simulink model "eVTOL_PX4_2023b"  (R2024b)
settings: Solver=ode4  StartTime=0  StopTime=inf  FixedStep=0.01  RelTol=1e-3
values from neighbouring files (symbols this model uses):
  aDl =     [initdata.mat]
  aDr =     [initdata.mat]
  aDyn =     [initdata.mat]
  Airport = init_airport('PHNL')    [initdata_HIL_eVTOL.m]
  aLat =     [initdata.mat]
  aLon =     [initdata.mat]
  D = Prop.D    [EOM_dt_MC.m]    (also in EOM_get_alf_dt_de_prop_evtol.m = CD * QS)
  dt0 = X(2)    [EOM_get_alf_dt_de_prop_evtol.m]    (also in initdata.mat = 0.258252593971; initdata_HIL_eVTOL.m = EOM_dt_MC)
  EAS0 = TAS0 / EAS2TAS    [initdata_HIL_eVTOL.m]
  FCS = init_FCS    [initdata_HIL_eVTOL.m]
  General = init_layoutdata    [EOM_dt_MC.m]    (also in build_optimized_CA.m; initdata.mat = ; initdata_HIL_eVTOL.m)
  h0 = Con(1)    [EOM_get_alf_dt_de_prop_evtol.m]    (also in initdata.mat = 450; initdata_HIL_eVTOL.m = 50)
  mass = Con(3)    [EOM_get_alf_dt_de_prop_evtol.m]    (also in initdata.mat = 2255.54; initdata_HIL_eVTOL.m = 7)
  Motor = init_motor_evtol    [EOM_dt_MC.m]    (also in initdata.mat = []; initdata_HIL_eVTOL.m)
  Prop = init_propeller_evtol_new    [EOM_dt_MC.m]    (also in initdata_HIL_eVTOL.m)
  R2D = 180/pi    (= 57.2957795131)    [EOM_get_alf_dt_de_prop_evtol.m]    (also in init_FCS.m; init_aerodata_evtol.m; init_airport.m; initdata.mat)
  SAMPLE_TIME = 0.01    [initdata_HIL_eVTOL.m]
  theta0 = -0.0510981441662    [initdata.mat]
undefined symbols (not defined in the file or in its folder): A1, aDa, aDe, aero, asbhl20env, B1, C1, de0, Earth, Environment, INIT_Data, InitData, Kd, Kp, magnitude, Newton, pProp, Raphson, Tc, WGS84
libraries: simulink_extras x63, vrlib x48, sharedtransform x28, simulink x22, slpidlib x20, sharedutil x20, matrix_library x18, aerolibwindfilters x12, aerolibobsolete x8, aerolibasang x8, aerolibatmos2 x6, aerolibfltsims x6
(part 7 of 17)

== system eVTOL_PX4_2023b/Subsystem2/Environment/Wind Models ==
  Xe_x : Inport
  Ve : Inport  Port=2
  Altitude : Inport  Port=3
  DCM : Inport  Port=4
  Constant1 : Constant  Value=[0,0,0]
  Constant2 : Constant  Value=[0,0,0]
  Dot Product1 : DotProduct  OutDataTypeStr=Inherit: Inherit via internal rule
  Dot Product2 : DotProduct  OutDataTypeStr=Inherit: Inherit via internal rule
  Dryden Wind Turbulence Model (Continuous (+q -r)) : Subsystem  AncestorBlock=|  mask(Wind Turbulence Model){units=Metric (MKS), spec=MIL-F-8785C, model=Continuous Dryden (+q -r), W20=8, Wdeg=0, TurbProb=10^-4, L_high=533.4, Wingspan=7, ts=0.01, Seed=[23341 23342 23343 23344], T_on=on}
      | CustomLib_2019b/Dryden Wind Turbulence Model 
      | (Continuous (+q -r))
      mask prompts: units "aeroblks:aeroblkwind:blockWindTurbulenceModelParamUnits"; spec "aeroblks:aeroblkwind:blockWindTurbulenceModelParamSpecification"; model "aeroblks:aeroblkwind:blockWindTurbulenceModelParamModeltype"; W20 "Wind speed at 6 m defines the low-altitude intensity (m/s):"; Wdeg "Wind direction at 6 m (degrees clockwise from north):"; TurbProb "aeroblks:aeroblkwind:blockWindTurbulenceModelParamProbabilityofexceedanceofhighaltitudeintensity"; L_high "Scale length at medium/high altitudes (m):"; Wingspan "Wingspan (m):"; ts "Band limited noise sample time (sec):"; Seed "aeroblks:aeroblkwind:blockWindTurbulenceModelParamNoiseseedsugvgwgpg"; T_on "aeroblks:aeroblkwind:blockWindTurbulenceModelParamTurbulenceon"
      mask help: aeroblks:aeroblkwind:blockWindTurbulenceModelDesc
      mask init: same as eVTOL_PX4_2023b/Subsystem1/Environment/Wind Models/Dryden Wind Turbulence Model (Continuous (+q -r))
      settings: LibrarySourceBlock=|
      | CustomLib_2019b/Dryden Wind Turbulence Model
      | (Continuous (+q -r))
      mask Help: eval('asbhelp(''Dryden Wind Turbulence Model (Continuous)'')');
      mask TypeOptions units: aeroblks:aeroblkwind:blockWindTurbulenceModelParamComboMetricMKS | aeroblks:aeroblkwind:blockWindTurbulenceModelParamComboEnglishVelocityinfts | aeroblks:aeroblkwind:blockWindTurbulenceModelParamComboEnglishVelocityinkts
      mask TypeOptions spec: aeroblks:aeroblkwind:blockWindTurbulenceModelParamComboMILF8785C | aeroblks:aeroblkwind:blockWindTurbulenceModelParamComboMILHDBK1797 | aeroblks:aeroblkwind:blockWindTurbulenceModelParamComboMILHDBK1797B
      mask TypeOptions model: aeroblks:aeroblkwind:blockWindTurbulenceModelParamComboContinuousVonKarmanqr1 | aeroblks:aeroblkwind:blockWindTurbulenceModelParamComboContinuousVonKarmanqr2 | aeroblks:aeroblkwind:blockWindTurbulenceModelParamComboContinuousVonKarmanqr3 | aeroblks:aeroblkwind:blockWindTurbulenceModelParamComboContinuousDrydenqr1 | aeroblks:aeroblkwind:blockWindTurbulenceModelParamComboContinuousDrydenqr2 | aeroblks:aeroblkwind:blockWindTurbulenceModelParamComboContinuousDrydenqr3 | aeroblks:aeroblkwind:blockWindTurbulenceModelParamComboDiscreteDrydenqr1 | aeroblks:aeroblkwind:blockWindTurbulenceModelParamComboDiscreteDrydenqr2 | aeroblks:aeroblkwind:blockWindTurbulenceModelParamComboDiscreteDrydenqr3
      mask Callback model: aeroicon('aeroblkwindturb2');
      mask TypeOptions TurbProb: aeroblks:aeroblkwind:blockWindTurbulenceModelParamCombo2x101 | aeroblks:aeroblkwind:blockWindTurbulenceModelParamCombo101 | aeroblks:aeroblkwind:blockWindTurbulenceModelParamCombo102Light | aeroblks:aeroblkwind:blockWindTurbulenceModelParamCombo103Moderate | aeroblks:aeroblkwind:blockWindTurbulenceModelParamCombo104 | aeroblks:aeroblkwind:blockWindTurbulenceModelParamCombo105Severe | aeroblks:aeroblkwind:blockWindTurbulenceModelParamCombo106
      mask DialogControl units Prompt: Units:
      mask DialogControl spec Prompt: Specification:
      mask DialogControl model Prompt: Model type:
      mask DialogControl TurbProb Prompt: Probability of exceedance of high-altitude intensity:
      mask DialogControl Seed Prompt: Noise seeds [ug vg wg pg]:
      mask DialogControl T_on Prompt: Turbulence on
      mask Display:
      | port_label(ports(1).type,ports(1).port,ports(1).txt,'texmode','on');
      | port_label(ports(2).type,ports(2).port,ports(2).txt,'texmode','on');
      | port_label(ports(3).type,ports(3).port,ports(3).txt,'texmode','on');
      | port_label(ports(4).type,ports(4).port,ports(4).txt,'texmode','on');
      | port_label(ports(5).type,ports(5).port,ports(5).txt,'texmode','on');
  Gain4 : Gain  Gain=[1,1,1]
  Manual Switch1 : ManualSwitch  CurrentSetting=0
  Manual Switch2 : ManualSwitch  CurrentSetting=0
  Sqrt : Sqrt
  vt1 : Math  Operator=sqrt  SignedPower=on
  wind scp2 : Scope
  wind_mag scp : Scope
  windangular scp : Scope
  windspeed scp : Scope
  ug,vg,wg1 : Outport  VectorParamsAs1DForOutWhenUnconnected=off
  pg,qg,rg1 : Outport  Port=2  VectorParamsAs1DForOutWhenUnconnected=off
  wires:
  Manual Switch2/1 -> ug,vg,wg1/1  "WindVelocity"
  Dryden Wind Turbulence Model (Continuous (+q -r))/1(ug,vg,wg) -> Gain4/1, windspeed scp/1, Dot Product2/2, Dot Product2/1  "Vw"
  Dryden Wind Turbulence Model (Continuous (+q -r))/2(pg,qg,rg) -> Manual Switch1/1, windangular scp/1  "WindAngularRates"
  Constant1/1 -> Manual Switch1/2
  Altitude/1 -> [Altitude]
  vt1/1 -> [Airspeed]  "Airspeed"
  Constant2/1 -> Manual Switch2/2
  [Airspeed] -> Dryden Wind Turbulence Model (Continuous (+q -r))/2(Airspeed)  "Airspeed"
  DCM/1 -> [DCM]
  Ve/1 -> Dot Product1/2, Dot Product1/1
  Manual Switch1/1 -> pg,qg,rg1/1  "WindAngularRates"
  Gain4/1 -> Manual Switch2/1  "WindVelocity"
  [Altitude] -> Dryden Wind Turbulence Model (Continuous (+q -r))/1(Altitude)
  Dot Product2/1 -> Sqrt/1
  [DCM] -> Dryden Wind Turbulence Model (Continuous (+q -r))/3(DCM)
  Dot Product1/1 -> vt1/1
  Sqrt/1 -> wind_mag scp/1  "wind_mag"
  Xe_x/1 -> [x]
  [x] -> wind scp2/1

== system eVTOL_PX4_2023b/Subsystem2/airframe/Flight Conditions ==
  EnvmData : Inport
  PlantData : Inport  Port=2
  Bus Selector1 : BusSelector  OutputSignals=WindVelocity,a,AirDensity,WindAngularRates,Po,To,g
  Bus Selector2 : BusSelector  OutputSignals=Xe,Ve,Vb,pqr,DCM_be
  Constant1 : Constant  Value=Airport.Elevation_m
  Constant2 : Constant  Value=1.225
  Demux : Demux  Outputs=2
  Derivative : Derivative  CoefficientInTFapproximation=100
  Divide : Product  Inputs=*/
  Divide1 : Product  Inputs=**
  Dynamic Pressure : aerolibasang/Dynamic Pressure
  Flat Earth to LLA1 : aerolibtransform2/Flat Earth to LLA  units=Metric (MKS)  ptype=Earth (WGS84)  F=1/298.257223563  R=6378137  refPosPort=off  LL0=InitData.LLA(1:2)*R2D  psi=0
  "Incidence, Sideslip, & Airspeed" : Subsystem  AncestorBlock=aerolibasang/Incidence, Sideslip, & Airspeed  mask(Incidence,Sideslip,&Airspeed){}
      mask help: Calculate the angles between the body and the velocity vector (incidence and sideslip), and the velocity magnitude from the components in body axes (Vb).
      settings: LibrarySourceBlock=|
      | aerolibasang/Incidence, Sideslip,
      | & Airspeed
      mask Help: web(asbhelp('incidence'));
      mask Display:
      | port_label('input',1,'V_b','texmode','on');
      | port_label('output',1,'\alpha','texmode','on');
      | port_label('output',2,'\beta','texmode','on');
      | port_label('output',3,'V','texmode','on');
  Mach Number : aerolibasang/Mach Number
  Product : Product  Multiplication=Matrix(*)
  Product1 : Product  Multiplication=Matrix(*)
  Sqrt : Sqrt
  Subsystem : Subsystem
  Sum1 : Sum  Inputs=+-|  InputSameDT=on  SaturateOnIntegerOverflow=on  OutDataTypeStr=Inherit: Same as first input
  Sum2 : Sum  Inputs=|+-  InputSameDT=on  SaturateOnIntegerOverflow=on  OutDataTypeStr=Inherit: Same as first input
  Terminator : Terminator
  Vw_b : Scope
  Vw_e : Scope
  lat_deg : Outport  VectorParamsAs1DForOutWhenUnconnected=off
  lon_deg : Outport  Port=2  VectorParamsAs1DForOutWhenUnconnected=off
  amsl : Outport  Port=3  VectorParamsAs1DForOutWhenUnconnected=off
  Alpha : Outport  Port=4  VectorParamsAs1DForOutWhenUnconnected=off
  AlphaDot : Outport  Port=5  VectorParamsAs1DForOutWhenUnconnected=off
  Beta : Outport  Port=6  VectorParamsAs1DForOutWhenUnconnected=off
  V : Outport  Port=7  VectorParamsAs1DForOutWhenUnconnected=off
  EAS : Outport  Port=8  VectorParamsAs1DForOutWhenUnconnected=off
  pqrWind : Outport  Port=9  VectorParamsAs1DForOutWhenUnconnected=off
  Mach : Outport  Port=10  VectorParamsAs1DForOutWhenUnconnected=off
  Qbar : Outport  Port=11  InitialOutput=0  VectorParamsAs1DForOutWhenUnconnected=off
  gamma : Outport  Port=12  InitialOutput=0  VectorParamsAs1DForOutWhenUnconnected=off
  chi : Outport  Port=13  InitialOutput=0  VectorParamsAs1DForOutWhenUnconnected=off
  Po : Outport  Port=14  VectorParamsAs1DForOutWhenUnconnected=off
  To : Outport  Port=15  VectorParamsAs1DForOutWhenUnconnected=off
  g : Outport  Port=16  VectorParamsAs1DForOutWhenUnconnected=off
  wires:
  Derivative/1 -> AlphaDot/1
  Bus Selector1/4 -> Product1/2  "<WindAngularRates>"
  Subsystem/1(gamma) -> gamma/1
  PlantData/1 -> Bus Selector2/1
  Sum2/1 -> "Incidence, Sideslip, & Airspeed"/1(Vb), Mach Number/1, Dynamic Pressure/1  "VA(b)"
  Subsystem/2(chi) -> chi/1
  Bus Selector2/3 -> Sum2/1  "<Vb>"
  Subsystem/3(V) -> Terminator/1
  Product1/1 -> Sum1/2
  Bus Selector1/5 -> Po/1  "<Po>"
  Mach Number/1 -> Mach/1  "Mach"
  "Incidence, Sideslip, & Airspeed"/1(Alpha) -> Derivative/1, Alpha/1  "Alpha"
  Product/1 -> Vw_b/1, Sum2/2
  Bus Selector2/2 -> Subsystem/1(<Ve>)  "<Ve>"
  "Incidence, Sideslip, & Airspeed"/2(Beta) -> Beta/1  "Beta"
  Dynamic Pressure/1 -> Qbar/1  "qbar"
  Bus Selector1/2 -> Mach Number/2  "<a>"
  Bus Selector2/5 -> Product/1, Product1/1  "<DCM_be>"
  Bus Selector2/4 -> Sum1/1  "<pqr>"
  Sum1/1 -> pqrWind/1
  EnvmData/1 -> Bus Selector1/1
  Bus Selector1/3 -> Divide/1, Dynamic Pressure/2  "<AirDensity>"
  Bus Selector1/1 -> Product/2, Vw_e/1  "<WindVelocity>"
  Bus Selector1/7 -> g/1  "<g>"
  Bus Selector1/6 -> To/1  "<To>"
  Demux/1 -> lat_deg/1  "lat_deg"
  Demux/2 -> lon_deg/1  "lon_deg"
  Flat Earth to LLA1/2 -> amsl/1  "amsl"
  Flat Earth to LLA1/1 -> Demux/1
  Constant1/1 -> Flat Earth to LLA1/2
  Bus Selector2/1 -> Flat Earth to LLA1/1  "<Xe>"
  Constant2/1 -> Divide/2
  Divide1/1 -> EAS/1
  Divide/1 -> Sqrt/1
  "Incidence, Sideslip, & Airspeed"/3(V) -> Divide1/1, V/1  "V"
  Sqrt/1 -> Divide1/2

== system eVTOL_PX4_2023b/Subsystem2/airframe/force moment ==
  note: force and moment in body fixed axis coordination
  PlantData : Inport
  Act_surface : Inport  Port=2
  prop : Inport  Port=3
  EnvmData : Inport  Port=4
  Add : Sum  Inputs=++++
  Add1 : Sum  Inputs=++++
  Disturbance : Constant  Value=[0,10,0]
  Disturbance1 : Constant  Value=[0,0,0]
  F_Gear_in_b scp : Scope  Commented=on
  Gear&FM in body axis : Subsystem  Commented=on
  M_Gear scp : Scope  Commented=on
  Manual Switch : ManualSwitch  CurrentSetting=0
  Motor moment scp : Scope
  Scope{,1..4,6} (6 alike) : Scope
  Thrust&M in body axis : Subsystem
  aero F&M in body axis : Subsystem
  gravity in body axis : Subsystem
  Fb (X Y Z) : Outport  VectorParamsAs1DForOutWhenUnconnected=off
  M (L M N) : Outport  Port=2  VectorParamsAs1DForOutWhenUnconnected=off
  wires:
  Thrust&M in body axis/1(f_T) -> Add/1, Scope4/1
  gravity in body axis/1(Fb) -> Add/3, Scope3/1
  Thrust&M in body axis/2(m_T) -> Add1/1, Motor moment scp/1
  aero F&M in body axis/2(M (L M N)) -> Scope6/1, Add1/2
  Add1/1 -> Scope1/1, M (L M N)/1
  Add/1 -> Scope/1, Fb (X Y Z)/1
  PlantData/1 -> aero F&M in body axis/1(PlantData), Gear&FM in body axis/1(PlantData), gravity in body axis/1(PlantData)
  Act_surface/1 -> aero F&M in body axis/2(Act_surface)
  EnvmData/1 -> gravity in body axis/2(EnvmData)
  Gear&FM in body axis/1(F_Gear) -> Add/4, F_Gear_in_b scp/1
  Gear&FM in body axis/2(M_Gear) -> Add1/3, M_Gear scp/1
  aero F&M in body axis/1(Fb (X Y Z)) -> Add/2, Scope2/1
  Disturbance/1 -> Manual Switch/1
  Manual Switch/1 -> Add1/4
  Disturbance1/1 -> Manual Switch/2
  prop/1 -> Thrust&M in body axis/1(prop)

== system eVTOL_PX4_2023b/UAV/Environment/Terrain ==
  Xe : Inport
  Terminator : Terminator
  hground_value : Constant  OutDataTypeStr=single
  hground : Outport  VectorParamsAs1DForOutWhenUnconnected=off
  wires:
  Xe/1 -> Terminator/1
  hground_value/1 -> hground/1  "hground"

== system eVTOL_PX4_2023b/UAV/Environment/Wind Models ==
  WindSpeed : Inport
  Ve : Inport  Port=2
  Altitude : Inport  Port=3
  DCM : Inport  Port=4
  Constant : Constant  Value=0
  Discrete Wind Gust Model1 : aerolibwind2/Discrete Wind Gust Model  units=Metric (MKS)  Gx=on  Gy=off  Gz=off  t_0=20  d_m=[10 10 6]*4  v_m=-[3.5 3.5 2.0]*1
  Discrete Wind Gust Model2 : aerolibwind2/Discrete Wind Gust Model  units=Metric (MKS)  Gx=on  Gy=off  Gz=off  t_0=28  d_m=[10 10 6]*4  v_m=[3.5 3.5 2.0]*1
  Dot Product : DotProduct  OutDataTypeStr=Inherit: Inherit via internal rule
  Gain : Gain
  Manual Switch : ManualSwitch
  Mux : Mux  Inputs=3
  Pulse Generator : DiscretePulseGenerator  PulseType=Time based  Amplitude=5  Period=1000  PulseWidth=99  PhaseDelay=1
  Sine Wave : Sin  Amplitude=0.2  SampleTime=0
  Sum : Sum  Inputs=+++++  InputSameDT=on  SaturateOnIntegerOverflow=on  OutDataTypeStr=Inherit: Same as first input
  Sum1 : Sum  Inputs=|++
  To Workspace8 : ToWorkspace  VariableName=VWindscp  SampleTime=-1
  Transform from Inertial to Body axes : Product  Inputs=**  Multiplication=Matrix(*)  InputSameDT=on  SaturateOnIntegerOverflow=on  OutDataTypeStr=Inherit: Same as first input
  constance wind : Constant  Value=[0, 2, 1]
  constance wind1 : Constant  Value=[0, 0, 0]
  constance wind2 : Constant  Value=[0, -2, 0]
  vt : Math  Operator=sqrt  SignedPower=on
  wind scp : Scope
  ug,vg,wg : Outport  VectorParamsAs1DForOutWhenUnconnected=off
  pg,qg,rg : Outport  Port=2  VectorParamsAs1DForOutWhenUnconnected=off
  wires:
  Ve/1 -> Dot Product/2, Dot Product/1
  Dot Product/1 -> vt/1
  vt/1 -> [Airspeed]  "Airspeed"
  Altitude/1 -> [Altitude]
  DCM/1 -> [DCM]
  Sum/1 -> To Workspace8/1, wind scp/1, ug,vg,wg/1  "WindVelocity"
  ? -> Sum/3
  [Airspeed] -> Discrete Wind Gust Model2/1, Discrete Wind Gust Model1/1  "Airspeed"
  constance wind1/1 -> pg,qg,rg/1  "WindAngularRates"
  [Altitude] -> ?
  [DCM] -> ?
  [Altitude] -> ?
  constance wind/1 -> ?
  [DCM] -> Transform from Inertial to Body axes/1
  Transform from Inertial to Body axes/1 -> Sum/1
  Constant/1 -> ?
  Mux/1 -> Manual Switch/2
  Manual Switch/1 -> Transform from Inertial to Body axes/2
  Sine Wave/1 -> Mux/3, Mux/2, Mux/1
  constance wind2/1 -> ?
  Discrete Wind Gust Model2/1 -> Sum1/2
  Sum1/1 -> Gain/1
  Discrete Wind Gust Model1/1 -> Sum1/1
  Gain/1 -> ?
  WindSpeed/1 -> Manual Switch/1

== system eVTOL_PX4_2023b/UAV/airframe/Flight Conditions ==
  EnvmData : Inport
  PlantData : Inport  Port=2
  Bus Selector1 : BusSelector  OutputSignals=WindVelocity,a,AirDensity,WindAngularRates,Po,To,g
  Bus Selector2 : BusSelector  OutputSignals=Xe,Ve,Vb,pqr
  Constant : Constant  Value=0
  Constant1 : Constant  Value=1.225
  Demux : Demux  Outputs=2
  Divide : Product  Inputs=*/
  Divide1 : Product  Inputs=**
  Dynamic Pressure : aerolibasang/Dynamic Pressure
  Flat Earth to LLA : aerolibtransform2/Flat Earth to LLA  units=Metric (MKS)  ptype=Earth (WGS84)  F=1/298.257223563  R=6378137  refPosPort=off  LL0=[INIT_Data.lat_deg, INIT_Data.lon_deg]  psi=0
  "Incidence, Sideslip, & Airspeed" : Subsystem  AncestorBlock=aerolibasang/Incidence, Sideslip, & Airspeed  mask(Incidence,Sideslip,&Airspeed){}
      mask help: Calculate the angles between the body and the velocity vector (incidence and sideslip), and the velocity magnitude from the components in body axes (Vb).
      mask Help: web(asbhelp('incidence'));
      mask Display:
      | port_label('input',1,'V_b','texmode','on');
      | port_label('output',1,'\alpha','texmode','on');
      | port_label('output',2,'\beta','texmode','on');
      | port_label('output',3,'V','texmode','on');
  Mach Number : aerolibasang/Mach Number
  Selector : Selector  InputPortWidth=3  IndexOptions=Index vector (dialog)  Indices=2  OutputSizes=1
  Sqrt : Sqrt
  Subsystem : Subsystem
  Sum1 : Sum  Inputs=++|  InputSameDT=on  SaturateOnIntegerOverflow=on  OutDataTypeStr=Inherit: Same as first input
  Sum2 : Sum  Inputs=|+-  InputSameDT=on  SaturateOnIntegerOverflow=on  OutDataTypeStr=Inherit: Same as first input
  Terminator : Terminator
  lat_deg : Outport  VectorParamsAs1DForOutWhenUnconnected=off
  lon_deg : Outport  Port=2  VectorParamsAs1DForOutWhenUnconnected=off
  amsl : Outport  Port=3  VectorParamsAs1DForOutWhenUnconnected=off
  Alpha : Outport  Port=4  VectorParamsAs1DForOutWhenUnconnected=off
  AlphaDot : Outport  Port=5  VectorParamsAs1DForOutWhenUnconnected=off
  Beta : Outport  Port=6  VectorParamsAs1DForOutWhenUnconnected=off
  V : Outport  Port=7  VectorParamsAs1DForOutWhenUnconnected=off
  EAS : Outport  Port=8  VectorParamsAs1DForOutWhenUnconnected=off
  pqrWind : Outport  Port=9  VectorParamsAs1DForOutWhenUnconnected=off
  Mach : Outport  Port=10  VectorParamsAs1DForOutWhenUnconnected=off
  Qbar : Outport  Port=11  InitialOutput=0  VectorParamsAs1DForOutWhenUnconnected=off
  gamma : Outport  Port=12  InitialOutput=0  VectorParamsAs1DForOutWhenUnconnected=off
  chi : Outport  Port=13  InitialOutput=0  VectorParamsAs1DForOutWhenUnconnected=off
  Po : Outport  Port=14  VectorParamsAs1DForOutWhenUnconnected=off
  To : Outport  Port=15  VectorParamsAs1DForOutWhenUnconnected=off
  g : Outport  Port=16  VectorParamsAs1DForOutWhenUnconnected=off
  wires:
  "Incidence, Sideslip, & Airspeed"/2(Beta) -> Beta/1  "Beta"
  "Incidence, Sideslip, & Airspeed"/3(V) -> Divide1/1, V/1  "V"
  Mach Number/1 -> Mach/1  "Mach"
  Dynamic Pressure/1 -> Qbar/1  "qbar"
  PlantData/1 -> Bus Selector2/1
  EnvmData/1 -> Bus Selector1/1
  Sum2/1 -> "Incidence, Sideslip, & Airspeed"/1(Vb), Mach Number/1, Dynamic Pressure/1  "VA(b)"
  Bus Selector2/3 -> Sum2/1  "<Vb>"
  Bus Selector1/1 -> Sum2/2  "<WindVelocity>"
  Bus Selector1/2 -> Mach Number/2  "<a>"
  Bus Selector1/3 -> [rho]  "<AirDensity>"
  Bus Selector1/4 -> Sum1/2  "<WindAngularRates>"
  Bus Selector2/4 -> [pqr]  "<pqr>"
  Sum1/1 -> pqrWind/1
  "Incidence, Sideslip, & Airspeed"/1(Alpha) -> Alpha/1  "Alpha"
  Selector/1 -> AlphaDot/1
  Bus Selector2/2 -> Subsystem/1(Xe)  "<Ve>"
  Subsystem/1(chi) -> chi/1
  Subsystem/2(gamma) -> gamma/1
  Subsystem/3(R) -> Terminator/1
  Bus Selector1/6 -> To/1  "<To>"
  Bus Selector1/5 -> Po/1  "<Po>"
  Bus Selector1/7 -> g/1  "<g>"
  Flat Earth to LLA/2 -> amsl/1  "amsl"
  Demux/1 -> lat_deg/1  "lat_deg"
  Demux/2 -> lon_deg/1  "lon_deg"
  Constant/1 -> Flat Earth to LLA/2
  Flat Earth to LLA/1 -> Demux/1
  Bus Selector2/1 -> Flat Earth to LLA/1  "<Xe>"
  [pqr] -> Sum1/1
  [pqr] -> Selector/1
  [rho] -> Dynamic Pressure/2
  [rho] -> Divide/1
  Constant1/1 -> Divide/2
  Divide/1 -> Sqrt/1
  Sqrt/1 -> Divide1/2
  Divide1/1 -> EAS/1

== system eVTOL_PX4_2023b/UAV/airframe/force moment ==
  note: force and moment in body fixed axis coordination
  PlantData : Inport
  ActData : Inport  Port=2
  EngineData_lo : Inport  Port=3
  EnvmData : Inport  Port=4
  Add : Sum  Inputs=++++
  Add1 : Sum  Inputs=++++
  Disturbance : Constant  Value=[0,10,0]
  Disturbance1 : Constant  Value=[0,0,0]
  F_Gear_in_b scp : Scope
  Gear&FM in body axis : Subsystem  Commented=on
  Gear&FM in body axis1 : Subsystem
  M_Gear scp : Scope
  Manual Switch : ManualSwitch  CurrentSetting=0
  Motor moment scp : Scope
  Scope{,1..4,6} (6 alike) : Scope
  Thrust in body axis1 : Subsystem
  aero F&M in body axis : Subsystem
  gravity in body axis : Subsystem
  Fb (X Y Z) : Outport  VectorParamsAs1DForOutWhenUnconnected=off
  M (L M N) : Outport  Port=2  VectorParamsAs1DForOutWhenUnconnected=off
  wires:
  Thrust in body axis1/1(f_T) -> Add/1, Scope4/1
  gravity in body axis/1(Fb) -> Add/3, Scope3/1
  Thrust in body axis1/2(m_T) -> Add1/1, Motor moment scp/1
  aero F&M in body axis/2(M (L M N)) -> Add1/2, Scope6/1
  Add1/1 -> M (L M N)/1, Scope1/1
  Add/1 -> Fb (X Y Z)/1, Scope/1
  PlantData/1 -> aero F&M in body axis/1(PlantData), Gear&FM in body axis1/1(PlantData), gravity in body axis/1(PlantData)
  ActData/1 -> aero F&M in body axis/2(ActData)
  EngineData_lo/1 -> Thrust in body axis1/1(EngineData)
  EnvmData/1 -> gravity in body axis/2(EnvmData)
  Gear&FM in body axis1/1(F_Gear) -> Add/4, F_Gear_in_b scp/1
  Gear&FM in body axis1/2(M_Gear) -> Add1/3, M_Gear scp/1
  aero F&M in body axis/1(Fb (X Y Z)) -> Add/2, Scope2/1
  Disturbance/1 -> Manual Switch/1
  Manual Switch/1 -> Add1/4
  Disturbance1/1 -> Manual Switch/2

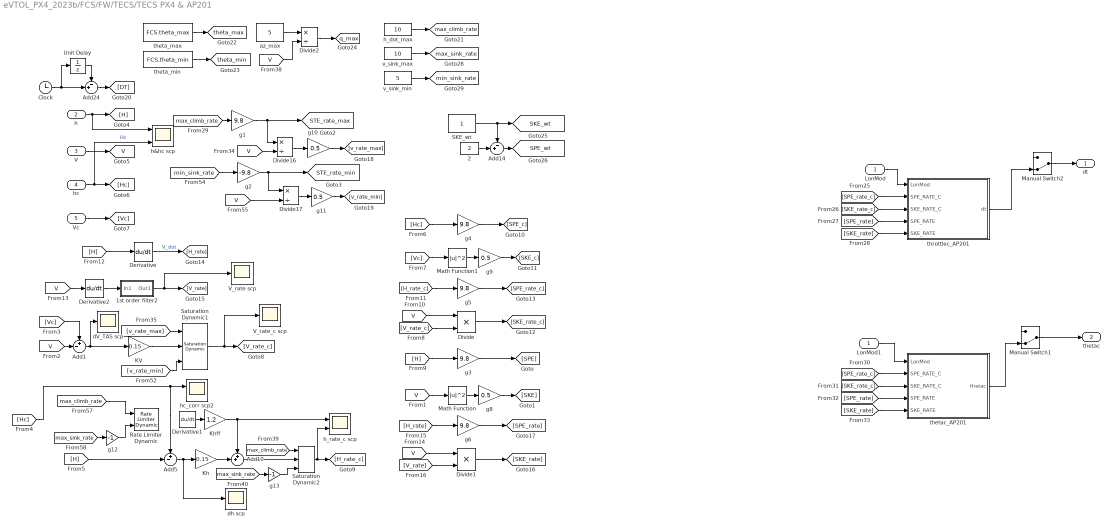
== system eVTOL_PX4_2023b/FCS/FW/TECS/TECS PX4 & AP201 ==
  LonMod : Inport
  h : Inport  Port=2
  V : Inport  Port=3
  hc : Inport  Port=4
  Vc : Inport  Port=5
  1st order filter2 : Subsystem
  2 : Constant  Value=2
  Add1 : Sum  Inputs=+-|
  Add10 : Sum  Inputs=++|
  Add14 : Sum  Inputs=-+|
  Add24 : Sum  Inputs=-+|
  Add5 : Sum  Inputs=+-|
  Clock : Clock
  Derivative : Derivative  CoefficientInTFapproximation=200
  Derivative1 : Derivative  CoefficientInTFapproximation=120
  Derivative2 : Derivative  CoefficientInTFapproximation=80
  Divide : Product  Inputs=**
  Divide1 : Product  Inputs=**
  Divide16 : Product  Inputs=*/
  Divide17 : Product  Inputs=*/
  Divide2 : Product  Inputs=*/
  KV : Gain  Gain=0.15
  Kh : Gain  Gain=0.15
  Khff : Gain  Gain=1.2
  LonMod1 : InportShadow
  Manual Switch1 : ManualSwitch  CurrentSetting=0
  Manual Switch2 : ManualSwitch  CurrentSetting=0
  Math Function : Math  Operator=magnitude^2  SignedPower=on
  Math Function1 : Math  Operator=magnitude^2  SignedPower=on
  Rate Limiter Dynamic : simulink/Discontinuities/Rate Limiter Dynamic
  SKE_wt : Constant
  Saturation Dynamic1 : simulink/Discontinuities/Saturation Dynamic  OutMin=[]  OutMax=[]  OutDataTypeStr=Inherit: Same as second input  OutDataType=fixdt(1, 16)  OutScaling=2^-10  DoSatur=off
  Saturation Dynamic2 : simulink/Discontinuities/Saturation Dynamic  OutMin=[]  OutMax=[]  OutDataTypeStr=Inherit: Same as second input  OutDataType=fixdt(1, 16)  OutScaling=2^-10  DoSatur=off
  Unit Delay : UnitDelay  SampleTime=-1  HasFrameUpgradeWarning=on
  V_rate scp : Scope
  V_rate_c scp : Scope
  az_max : Constant  Value=5
  dV_TAS scp : Scope
  dh scp : Scope
  g{1,3..6} (5 alike) : Gain  Gain=9.8
  g{8..11} (4 alike) : Gain  Gain=0.5
  g12 : Gain  Gain=-1
  g13 : Gain  Gain=-1
  g2 : Gain  Gain=-9.8
  h&hc scp : Scope  NumInputPorts=2
  h_dot_max : Constant  Value=10
  h_rate_c scp : Scope  NumInputPorts=2
  hc_corr scp2 : Scope  NumInputPorts=2
  theta_max : Constant  Value=FCS.theta_max
  theta_min : Constant  Value=FCS.theta_min
  thetac_AP201 : Subsystem
  throttlec_AP201 : Subsystem
  v_sink_max : Constant  Value=10
  v_sink_min : Constant  Value=5
  dt : Outport  VectorParamsAs1DForOutWhenUnconnected=off
  thetac : Outport  Port=2  VectorParamsAs1DForOutWhenUnconnected=off
  tag scope: SKE_wt=global, SPE_wt=global, STE_rate_max=global, STE_rate_min=global, V=global, max_climb_rate=global, max_sink_rate=global, min_sink_rate=global, q_max=global, theta_max=global, theta_min=global
  wires:
  Vc/1 -> [Vc]
  V/1 -> [V]
  h/1 -> h&hc scp/1, [H]
  Math Function/1 -> g8/1
  g3/1 -> [SPE]
  hc/1 -> h&hc scp/2, [Hc]  "Hc"
  [H] -> g3/1
  [V] -> Math Function/1
  [V] -> Add1/2
  [Vc] -> Add1/1
  Saturation Dynamic1/1 -> V_rate_c scp/1, [V_rate_c]
  [H] -> Add5/2
  Derivative1/1 -> Khff/1
  Kh/1 -> Add10/2
  Khff/1 -> Add10/1, h_rate_c scp/1
  Saturation Dynamic2/1 -> h_rate_c scp/2, [H_rate_c]
  [Hc] -> g4/1
  g4/1 -> [SPE_c]
  [Vc] -> Math Function1/1
  Math Function1/1 -> g9/1
  [V] -> Divide/1
  [V_rate_c] -> Divide/2
  Divide/1 -> [SKE_rate_c]
  [H_rate_c] -> g5/1
  g5/1 -> [SPE_rate_c]
  [H] -> Derivative/1
  Derivative/1 -> [H_rate]  "V_dot"
  [V] -> Derivative2/1
  1st order filter2/1(Out1) -> V_rate scp/1, [V_rate]
  g6/1 -> [SPE_rate]
  [H_rate] -> g6/1
  Divide1/1 -> [SKE_rate]
  [V_rate] -> Divide1/2
  [V] -> Divide1/1
  SKE_wt/1 -> Add14/1, [SKE_wt]
  2/1 -> Add14/2
  Add14/1 -> [SPE_wt]
  Add5/1 -> dh scp/1, Kh/1
  g8/1 -> [SKE]
  g9/1 -> [SKE_c]
  Add1/1 -> KV/1, dV_TAS scp/1
  KV/1 -> Saturation Dynamic1/2
  [v_rate_max] -> Saturation Dynamic1/1
  [v_rate_min] -> Saturation Dynamic1/3
  [Hc] -> Add5/1, hc_corr scp2/1
  [max_climb_rate] -> Rate Limiter Dynamic/1
  [max_sink_rate] -> g12/1
  theta_max/1 -> [theta_max]
  theta_min/1 -> [theta_min]
  Divide2/1 -> [q_max]
  Derivative2/1 -> 1st order filter2/1(In1)
  v_sink_max/1 -> [max_sink_rate]
  [min_sink_rate] -> g2/1
  [max_climb_rate] -> g1/1
  Divide16/1 -> g10/1
  [V] -> Divide16/2
  g2/1 -> Divide17/1, [STE_rate_min]
  v_sink_min/1 -> [min_sink_rate]
  g10/1 -> [v_rate_max]
  g1/1 -> Divide16/1, [STE_rate_max]
  g11/1 -> [v_rate_min]
  [V] -> Divide17/2
  Divide17/1 -> g11/1
  Clock/1 -> Unit Delay/1, Add24/2
  Add24/1 -> [DT]
  Unit Delay/1 -> Add24/1
  throttlec_AP201/1(dt) -> Manual Switch2/2
  Manual Switch2/1 -> dt/1
  thetac_AP201/1(thetac) -> Manual Switch1/2
  [SPE_rate_c] -> throttlec_AP201/2(SPE_RATE_C)
  [SKE_rate_c] -> throttlec_AP201/3(SKE_RATE_C)
  [SPE_rate] -> throttlec_AP201/4(SPE_RATE)
  [SKE_rate] -> throttlec_AP201/5(SKE_RATE)
  [SPE_rate_c] -> thetac_AP201/2(SPE_RATE_C)
  [SKE_rate_c] -> thetac_AP201/3(SKE_RATE_C)
  [SPE_rate] -> thetac_AP201/4(SPE_RATE)
  [SKE_rate] -> thetac_AP201/5(SKE_RATE)
  Manual Switch1/1 -> thetac/1
  az_max/1 -> Divide2/1
  [V] -> Divide2/2
  h_dot_max/1 -> [max_climb_rate]
  g12/1 -> Rate Limiter Dynamic/3
  Add10/1 -> Saturation Dynamic2/2
  [max_climb_rate] -> Saturation Dynamic2/1
  [max_sink_rate] -> g13/1
  g13/1 -> Saturation Dynamic2/3
  LonMod/1 -> throttlec_AP201/1(LonMod)
  LonMod1/1 -> thetac_AP201/1(LonMod)

== system eVTOL_PX4_2023b/FCS/FW/V hold//control/Subsystem3 ==
  VMod : Inport
  dvbar : Inport  Port=2
  Add1 : Sum  Commented=on  Inputs=+++
  Data Type Conversion : DataTypeConversion  OutDataTypeStr=boolean  SaturateOnIntegerOverflow=off  RndMeth=Floor
  Derivative : Derivative  Commented=on  CoefficientInTFapproximation=100
  Detect Change : simulink/Logic and Bit Operations/Detect Change  Commented=on  vinit=0  OutDataTypeStr=boolean
  Integrator : Integrator  Commented=on  ExternalReset=either  LimitOutput=on  UpperSaturationLimit=0.5  LowerSaturationLimit=-0.5
  KV : Gain  Commented=on  Gain=5
  KVD : Gain  Commented=on  Gain=5
  "KVi " : Gain  Commented=on  Gain=0.5
  KVi 1 : Gain  Commented=on  Gain=-1
  Memory : Memory
  PID Controller : slpidlib/PID Controller  Controller=PID  Form=Parallel  TimeDomain=Continuous-time  UseExternalTs=off  SampleTime=-1  IntegratorMethod=Forward Euler  FilterMethod=Forward Euler  ControllerParametersSource=internal  P=-5  I=-0.5  UseKiTs=off  D=-5  N=100  UseFilter=on  TunerSelectOption=Transfer Function Based (PID Tuner App)  InitialConditionSource=internal  InitialConditionForIntegrator=0  InitialConditionForFilter=0  DifferentiatorICPrevScaledInput=0  ExternalReset=rising  TrackingMode=off  Kt=1  LimitOutput=on  SatLimitsSource=internal  UpperSaturationLimit=1  LowerSaturationLimit=0  LinearizeAsGain=on  AntiWindupMode=clamping  Kb=1  LimitIntegrator=off  UpperIntegratorSaturationLimit=inf  LowerIntegratorSaturationLimit=-inf  POutMin=[]  POutMax=[]  IOutMin=[]  IOutMax=[]  DOutMin=[]  DOutMax=[]  NOutMin=[]  NOutMax=[]  SumOutMin=[]  SumOutMax=[]  SaturationOutMin=[]  SaturationOutMax=[]  PParamMin=[]  PParamMax=[]  IParamMin=[]  IParamMax=[]  DParamMin=[]  DParamMax=[]  NParamMin=[]  NParamMax=[]  KbParamMin=[]  KbParamMax=[]  KtParamMin=[]  KtParamMax=[]  KbOutMin=[]  KbOutMax=[]  KtOutMin=[]  KtOutMax=[]  IntegratorOutMin=[]  IntegratorOutMax=[]  FilterOutMin=[]  FilterOutMax=[]  SumI1OutMin=[]  SumI1OutMax=[]  SumI2OutMin=[]  SumI2OutMax=[]  SumI3OutMin=[]  SumI3OutMax=[]  SumI4OutMin=[]  SumI4OutMax=[]  SumDOutMin=[]  SumDOutMax=[]  DifferentiatorOutMin=[]  DifferentiatorOutMax=[]  FilterDiffOutCoefMin=[]  FilterDiffOutCoefMax=[]  ReciprocalOutMin=[]  ReciprocalOutMax=[]  SumDenOutMin=[]  SumDenOutMax=[]  SumNumOutMin=[]  SumNumOutMax=[]  DivideOutMin=[]  DivideOutMax=[]  UdiffTsProdOutMin=[]  UdiffTsProdOutMax=[]  NTsProdOutMin=[]  NTsProdOutMax=[]  UintegralTsProdOutMin=[]  UintegralTsProdOutMax=[]  UngainTsProdOutMin=[]  UngainTsProdOutMax=[]  ClampingZeroOutDataTypeStr=Inherit: Inherit via back propagation  ClampingZeroOutMin=[]  ClampingZeroOutMax=[]  FilterDenConstantOutDataTypeStr=Inherit: Inherit via back propagation  FilterDenConstantOutMin=[]  FilterDenConstantOutMax=[]  PCopyOutDataTypeStr=Inherit: Inherit via back propagation  PCopyOutMin=[]  PCopyOutMax=[]  NCopyOutDataTypeStr=Inherit: Inherit via back propagation  NCopyOutMin=[]  NCopyOutMax=[]  IntegratorContinuousStateAttributes=''  IntegratorStateMustResolveToSignalObject=off  IntegratorRTWStateStorageClass=Auto  FilterContinuousStateAttributes=''  FilterStateMustResolveToSignalObject=off  FilterRTWStateStorageClass=Auto  ParallelPVariant=InternalParameters  IdealPVariant=Disabled  IVariant=InternalParameters  DVariant=InternalParameters  IntegratorVariant=Continuous  SatVariant=Enabled  AWVariant=ContClampingParallel  PCopyVariant=Disabled  TRVariant=Disabled  FdbkBlocksVariant=Forward  IdealPFdbkVariant=Disabled  SatFdbkVariant=Disabled  DerivativeFilterVariant=ContFilter  NVariant=InternalParameters  NCopyVariant=Disabled  FilterICVariant=InternalICsFilter  IntegratorICVariant=InternalICs  ExternalResetVariant=ExternalReset  TRSumVariant=Passthrough  SumFdbkVariant=Disabled  SumVariant=Sum_PID  TsampFilterVariant=InternalTs  TsampNgainVariant=Passthrough  TsampIntegralVariant=Disabled_SignalSpec  ExternalSaturationOutDataTypeStr=Inherit: Same as second input
  Product2 : Product  RndMeth=Zero
  dvbar scp : Scope
  dt_cmd : Outport  VectorParamsAs1DForOutWhenUnconnected=off
  wires:
  dvbar/1 -> Product2/2
  Integrator/1 -> "KVi "/1
  "KVi "/1 -> Add1/1
  KV/1 -> Add1/2
  Add1/1 -> KVi 1/1
  KVD/1 -> ?
  Derivative/1 -> KVD/1
  Product2/1 -> dvbar scp/1, PID Controller/1
  PID Controller/1 -> dt_cmd/1
  VMod/1 -> Memory/1, Product2/1
  Memory/1 -> Data Type Conversion/1
  Data Type Conversion/1 -> PID Controller/2

== system eVTOL_PX4_2023b/FCS/FW/V hold//control/dt Fade at 0.1 // sec ==
  dt_ini : Inport
  Enable : EnablePort
  Chart : Stateflow chart  TreatAsAtomicUnit=on
  Constant : Constant
  Gain : Gain  Gain=0.1
  Integrator : Integrator
  Sum : Sum  Inputs=|+-
  dt_Out : Outport  VectorParamsAs1DForOutWhenUnconnected=off
  wires:
  Integrator/1 -> Sum/2
  Gain/1 -> Integrator/1
  Constant/1 -> Gain/1
  Sum/1 -> dt_Out/1
  Chart/1(dt) -> Sum/1
  dt_ini/1 -> Chart/1(dt_ini)

== system eVTOL_PX4_2023b/FCS/FW/V hold//control/getV_bar ==
  V : Inport
  V_c : Inport  Port=2
  Divide : Product  Inputs=*/
  Saturation1 : Saturate  UpperLimit=300  LowerLimit=0.1
  Saturation2 : Saturate  UpperLimit=1/3  LowerLimit=-1/3
  Sum : Sum  Inputs=+-
  dv scp : Scope
  V_bar : Outport  InitialOutput=0  VectorParamsAs1DForOutWhenUnconnected=off
  wires:
  Saturation2/1 -> V_bar/1
  Saturation1/1 -> Divide/2, Sum/2
  Divide/1 -> Saturation2/1
  Sum/1 -> Divide/1, dv scp/1
  V_c/1 -> Saturation1/1
  V/1 -> Sum/1

== system eVTOL_PX4_2023b/FCS/FW/alpha limit/Subsystem ==
  In1 : Inport
  Enable : EnablePort
  Out1 : Outport  VectorParamsAs1DForOutWhenUnconnected=off
  wires:
  In1/1 -> Out1/1

== system eVTOL_PX4_2023b/FCS/MC/ADRC theta/ESO ==
  u : Inport
  x0 : Inport  Port=2
  Gain : Gain  Gain=A1  Multiplication=Matrix(K*u)
  Gain1 : Gain  Gain=B1  Multiplication=Matrix(K*u)
  Gain2 : Gain  Gain=C1  Multiplication=Matrix(K*u)
  Integrator : Integrator  InitialConditionSource=external  InitialCondition=[pi/4, 0, 0]
  Sum : Sum  Inputs=|++
  x : Outport
  y : Outport  Port=2
  wires:
  Integrator/1 -> Gain/1, Gain2/1, x/1  "x"
  u/1 -> Gain1/1
  Gain/1 -> Sum/1
  Gain1/1 -> Sum/2
  Gain2/1 -> y/1
  Sum/1 -> Integrator/1  "x_dot"
  x0/1 -> Integrator/2

== system eVTOL_PX4_2023b/FCS/MC/ADRC theta/TD ==
  v : Inport
  Product : Product
  Product1 : Product
  Sum : Sum  Inputs=|++
  Sum1 : Sum  Inputs=|+-
  Sum2 : Sum  Inputs=++|
  Unit Delay : UnitDelay  InitialCondition=pi/4  SampleTime=-1  HasFrameUpgradeWarning=on
  Unit Delay1 : UnitDelay  SampleTime=-1  HasFrameUpgradeWarning=on
  fhan : Subsystem
  h : Constant  Value=0.01
  r : Constant  Value=0.3
  v1 : Outport
  v2 : Outport  Port=2
  wires:
  [v] -> Sum1/2
  Sum1/1 -> fhan/1(x1)
  Unit Delay1/1 -> Sum2/1, Product/2, [x2_k], fhan/2(x2)  "x2(k)"
  h/1 -> [h]
  Unit Delay/1 -> Sum/1, [x1_k]  "x1(k)"
  Product1/1 -> Sum2/2
  r/1 -> fhan/3(r)
  Sum2/1 -> Unit Delay1/1  "x2(k+1)"
  [h] -> fhan/4(h)
  fhan/1(fhan) -> Product1/2  "fh"
  [h] -> Product/1
  [h] -> Product1/1
  [x1_k] -> Sum1/1
  v/1 -> [v]
  Product/1 -> Sum/2
  Sum/1 -> Unit Delay/1  "x1(k+1)"
  [x1_k] -> v1/1
  [x2_k] -> v2/1

== system eVTOL_PX4_2023b/FCS/MC/ADRC theta/consituous TD ==
  v : Inport
  Derivative : Derivative
  Linear Second-Order Actuator : aerolibactuator/Linear Second-Order Actuator  wn_fin=3  z_fin=0.9  fin_act_0=pi/4  fin_act_vel=0
  TD : TransferFcn  Commented=on  Numerator=[1, 0]  Denominator=[Tc^2, 2*Tc, 1]
  v1 : Outport
  v2 : Outport  Port=2
  wires:
  Linear Second-Order Actuator/1 -> TD/1, Derivative/1, v1/1
  TD/1 -> v2/1  "r_dot"
  v/1 -> Linear Second-Order Actuator/1

== system eVTOL_PX4_2023b/Subsystem1/Energy & Power/V_prop1/v_b to v_prop ==
  V_body : Inport
  i : Inport  Port=2
  Add : Sum  Inputs=+-
  Mux1 : Mux  Inputs=2
  Terminator : Terminator
  V_x : Fcn  Expr=u[1]*cos(u[4])
  V_y : Fcn  Expr=0
  V_z : Fcn  Expr=u[3]*sin(u[4])
  V : Outport  VectorParamsAs1DForOutWhenUnconnected=off
  wires:
  i/1 -> Mux1/2
  V_body/1 -> Mux1/1
  Mux1/1 -> V_z/1, V_y/1, V_x/1
  Add/1 -> V/1
  V_x/1 -> Add/1
  V_z/1 -> Add/2
  V_y/1 -> Terminator/1

== system eVTOL_PX4_2023b/Subsystem1/Energy & Power/V_prop2/v_b to v_prop ==
  V_body : Inport
  i : Inport  Port=2
  Add : Sum  Inputs=+-
  Mux1 : Mux  Inputs=2
  Terminator : Terminator
  V_x : Fcn  Expr=u[1]*cos(u[4])
  V_y : Fcn  Expr=0
  V_z : Fcn  Expr=u[3]*sin(u[4])
  V : Outport  VectorParamsAs1DForOutWhenUnconnected=off
  wires:
  i/1 -> Mux1/2
  V_body/1 -> Mux1/1
  Mux1/1 -> V_z/1, V_y/1, V_x/1
  V_z/1 -> Add/2
  V_x/1 -> Add/1
  Add/1 -> V/1
  V_y/1 -> Terminator/1

== system eVTOL_PX4_2023b/Subsystem1/Energy & Power/V_prop3/v_b to v_prop ==
  V_body : Inport
  i : Inport  Port=2
  Add : Sum  Inputs=+-
  Mux1 : Mux  Inputs=2
  Terminator : Terminator
  V_x : Fcn  Expr=u[1]*cos(u[4])
  V_y : Fcn  Expr=0
  V_z : Fcn  Expr=u[3]*sin(u[4])
  V : Outport  VectorParamsAs1DForOutWhenUnconnected=off
  wires:
  i/1 -> Mux1/2
  V_body/1 -> Mux1/1
  Mux1/1 -> V_z/1, V_y/1, V_x/1
  V_z/1 -> Add/2
  V_x/1 -> Add/1
  Add/1 -> V/1
  V_y/1 -> Terminator/1

== system eVTOL_PX4_2023b/Subsystem1/Energy & Power/V_prop4/v_b to v_prop ==
  V_body : Inport
  i : Inport  Port=2
  Add : Sum  Inputs=+-
  Mux1 : Mux  Inputs=2
  Terminator : Terminator
  V_x : Fcn  Expr=u[1]*cos(u[4])
  V_y : Fcn  Expr=0
  V_z : Fcn  Expr=u[3]*sin(u[4])
  V : Outport  VectorParamsAs1DForOutWhenUnconnected=off
  wires:
  i/1 -> Mux1/2
  V_body/1 -> Mux1/1
  Mux1/1 -> V_z/1, V_y/1, V_x/1
  V_x/1 -> Add/1
  Add/1 -> V/1
  V_z/1 -> Add/2
  V_y/1 -> Terminator/1

== system eVTOL_PX4_2023b/Subsystem1/Energy & Power/V_prop5/v_b to v_prop ==
  V_body : Inport
  i : Inport  Port=2
  Add : Sum  Inputs=+-
  Mux1 : Mux  Inputs=2
  Terminator : Terminator
  V_x : Fcn  Expr=u[1]*cos(u[4])
  V_y : Fcn  Expr=0
  V_z : Fcn  Expr=u[3]*sin(u[4])
  V : Outport  VectorParamsAs1DForOutWhenUnconnected=off
  wires:
  i/1 -> Mux1/2
  V_body/1 -> Mux1/1
  Mux1/1 -> V_z/1, V_y/1, V_x/1
  V_z/1 -> Add/2
  V_x/1 -> Add/1
  Add/1 -> V/1
  V_y/1 -> Terminator/1

== system eVTOL_PX4_2023b/Subsystem1/Energy & Power/V_prop6/v_b to v_prop ==
  V_body : Inport
  i : Inport  Port=2
  Add : Sum  Inputs=+-
  Mux1 : Mux  Inputs=2
  Terminator : Terminator
  V_x : Fcn  Expr=u[1]*cos(u[4])
  V_y : Fcn  Expr=0
  V_z : Fcn  Expr=u[3]*sin(u[4])
  V : Outport  VectorParamsAs1DForOutWhenUnconnected=off
  wires:
  i/1 -> Mux1/2
  V_body/1 -> Mux1/1
  Mux1/1 -> V_z/1, V_y/1, V_x/1
  V_z/1 -> Add/2
  V_x/1 -> Add/1
  Add/1 -> V/1
  V_y/1 -> Terminator/1

== system eVTOL_PX4_2023b/Subsystem1/Energy & Power/thrust_1/Motor ==
  P_shaft : Inport
  dt : Inport  Port=2
  V : Inport  Port=3
  rpm0 : Inport  Port=4
  rho : Inport  Port=5
  theta_b : Inport  Port=6
  Add : Sum
  Constant : Constant  Value=Motor.Ue
  Constant1 : Constant  Value=Motor.Re
  Constant2 : Constant  Value=Motor.Rm
  Constant3 : Constant  Value=Motor.KE
  Constant4 : Constant  Value=Motor.KT  VectorParams1D=off
  Constant5 : Constant  Value=Motor.Im0
  Constant6 : Constant  Value=0
  Constant7 : Constant  Value=0.001
  D^5 : Constant  Value=5
  Diameter : Constant  Value=Prop.D
  Diameter1 : Constant  Value=Prop.D
  Divide : Product  Inputs=*//
  Ea : Sum  Inputs=+-
  Gain1 : Gain  Gain=30/pi
  Gain2 : Gain  Gain=pi/30
  Gain3 : Gain  Gain=1/60
  Gain4 : Gain  Gain=1/(2*pi)
  Im : Sum
  Integrator : Integrator  InitialConditionSource=external  InitialCondition=600
  Ix : Constant  Value=Prop.Ix/8
  J : Product  Inputs=*//
  Manual Switch : ManualSwitch
  Math Function : Math  Operator=magnitude^2  SignedPower=on
  Math Function3 : Math  Operator=pow  SignedPower=on
  Math Function4 : Math  Operator=pow  SignedPower=on
  Memory : Memory  InitialCondition=0.1
  N(rpm) : Product  Inputs=*/
  N(rpm)1 : Product  Inputs=/*
  P Scope : Scope  NumInputPorts=2
  P_sp : Product  Inputs=4
  Product1 : Product
  Product2 : Product
  Q : Product  Inputs=4
  RPM 1 : Scope  NumInputPorts=2
  Saturation : Saturate  UpperLimit=104.72  LowerLimit=0.1
  Scope : Scope
  Sum : Sum  Inputs=|+-
  Ueo : Product
  Um : Sum  Inputs=+-
  get CP : Lookup_n-D  BreakpointsForDimension1=Prop.J  BreakpointsForDimension2=Prop.theta_b  IndexSearchMethod=Linear search  BeginIndexSearchUsingPreviousIndexResult=on  Table=Prop.CP  RndMeth=Simplest
      settings: InputPortMap=u0,u1
  "n^3 " : Constant  Value=3
  rpm : Outport  VectorParamsAs1DForOutWhenUnconnected=off
  wires:
  Saturation/1 -> Gain1/1, Divide/2
  Gain2/1 -> Integrator/2
  rpm0/1 -> Manual Switch/1
  Gain1/1 -> rpm/1, RPM 1/1  "rpm"
  Sum/1 -> Divide/1  "DP"
  Divide/1 -> Integrator/1  "omega_dot"
  Integrator/1 -> Saturation/1  "omega"
  P_sp/1 -> Scope/1, P Scope/1, Sum/1
  P_shaft/1 -> P Scope/2, Sum/2
  Ix/1 -> Divide/3
  Constant/1 -> Ueo/2
  Ueo/1 -> Um/1
  Product1/1 -> Um/2
  Constant1/1 -> Product1/1
  Um/1 -> Ea/1
  Product2/1 -> Ea/2
  Constant2/1 -> Product2/1
  Ea/1 -> N(rpm)/1
  Constant3/1 -> N(rpm)/2
  Diameter/1 -> J/2
  V/1 -> J/1
  N(rpm)/1 -> Gain3/1, RPM 1/2
  J/1 -> get CP/1
  theta_b/1 -> get CP/2
  Gain4/1 -> Q/2  "CQ"
  D^5/1 -> Math Function4/2
  Diameter1/1 -> Math Function4/1
  Math Function/1 -> Q/3  "n^2"
  Q/1 -> N(rpm)1/2
  Constant4/1 -> N(rpm)1/1
  N(rpm)1/1 -> Im/1
  Constant5/1 -> Im/2
  Im/1 -> Product2/2, Product1/2
  rho/1 -> Q/1, P_sp/3  "rho"
  Math Function3/1 -> P_sp/2  "n^3"
  "n^3 "/1 -> Math Function3/2
  Math Function4/1 -> Q/4, P_sp/4  "D^5"
  get CP/1 -> Gain4/1, P_sp/1  "CP"
  Manual Switch/1 -> Gain2/1
  Constant6/1 -> Manual Switch/2
  Constant7/1 -> Add/1
  Add/1 -> Ueo/1
  dt/1 -> Add/2
  Gain3/1 -> Memory/1  "rps"
  Memory/1 -> J/3, Math Function3/1, Math Function/1

== system eVTOL_PX4_2023b/Subsystem1/Energy & Power/thrust_1/Propeller  ==
  rpm : Inport
  V : Inport  Port=2
  rho : Inport  Port=3
  theta_b : Inport  Port=4
  D^5 : Constant  Value=5
  Diameter : Constant  Value=Prop.D
  Display1 : Display
  Display7 : Display
  Divide : Product  Inputs=4
  Divide2 : Product  Inputs=4
  Divide3 : Product  Inputs=**/
  Gain : Gain  Gain=1/60
  Math Function : Math  Operator=magnitude^2  SignedPower=on
  Math Function1 : Math  Operator=magnitude^2  SignedPower=on
  Math Function2 : Math  Operator=magnitude^2  SignedPower=on
  Math Function3 : Math  Operator=pow  SignedPower=on
  Math Function4 : Math  Operator=pow  SignedPower=on
  Scope{,1..4} (5 alike) : Scope
  Subsystem : Subsystem
  get CP : Lookup_n-D  BreakpointsForDimension1=Prop.J  BreakpointsForDimension2=Prop.theta_b  IndexSearchMethod=Linear search  BeginIndexSearchUsingPreviousIndexResult=on  Table=Prop.CP  RndMeth=Simplest
      settings: InputPortMap=u0,u1
  get CT : Lookup_n-D  BreakpointsForDimension1=Prop.J  BreakpointsForDimension2=Prop.theta_b  IndexSearchMethod=Linear search  BeginIndexSearchUsingPreviousIndexResult=on  Table=Prop.CT  RndMeth=Simplest
      settings: InputPortMap=u0,u1
  "n^3 " : Constant  Value=3
  P_plr (w) : Outport  VectorParamsAs1DForOutWhenUnconnected=off
  T (N) : Outport  Port=2  VectorParamsAs1DForOutWhenUnconnected=off
  eta_p : Outport  Port=3  VectorParamsAs1DForOutWhenUnconnected=off
  wires:
  Divide2/1 -> Scope/1, P_plr (w)/1
  Divide3/1 -> eta_p/1  "eta_p"
  D^5/1 -> Math Function4/2
  Math Function4/1 -> Divide2/4
  "n^3 "/1 -> Math Function3/2
  Math Function3/1 -> Divide2/3
  get CP/1 -> Display1/1, Divide3/3, Divide2/1, Scope3/1
  rpm/1 -> Gain/1, Subsystem/2(rpm)
  Subsystem/1(J) -> Scope2/1, get CT/1, Divide3/1, get CP/1
  Divide/1 -> Scope1/1, T (N)/1
  Math Function2/1 -> Divide/4  "D^4"
  Math Function1/1 -> Math Function2/1
  Diameter/1 -> Math Function1/1, Math Function4/1
  Math Function/1 -> Divide/3  "n^2"
  Gain/1 -> Math Function3/1, Math Function/1
  rho/1 -> Divide/2, Divide2/2
  get CT/1 -> Display7/1, Divide3/2, Divide/1, Scope4/1
  V/1 -> Subsystem/1(V)
  theta_b/1 -> get CP/2, get CT/2

== system eVTOL_PX4_2023b/Subsystem1/Energy & Power/thrust_2/Motor ==
  P_shaft : Inport
  dt : Inport  Port=2
  V : Inport  Port=3
  rpm0 : Inport  Port=4
  rho : Inport  Port=5
  theta_b : Inport  Port=6
  Constant : Constant  Value=Motor.Ue
  Constant1 : Constant  Value=Motor.Re
  Constant2 : Constant  Value=Motor.Rm
  Constant3 : Constant  Value=Motor.KE
  Constant4 : Constant  Value=Motor.KT  VectorParams1D=off
  Constant5 : Constant  Value=Motor.Im0
  Constant6 : Constant  Value=0
  D^5 : Constant  Value=5
  Diameter : Constant  Value=Prop.D
  Diameter1 : Constant  Value=Prop.D
  Divide : Product  Inputs=*//
  Ea : Sum  Inputs=+-
  Gain1 : Gain  Gain=30/pi
  Gain2 : Gain  Gain=pi/30
  Gain3 : Gain  Gain=1/60
  Gain4 : Gain  Gain=1/(2*pi)
  Im : Sum
  Integrator : Integrator  InitialConditionSource=external  InitialCondition=600
  Ix : Constant  Value=Prop.Ix/8
  J : Product  Inputs=*//
  Manual Switch : ManualSwitch
  Math Function : Math  Operator=magnitude^2  SignedPower=on
  Math Function3 : Math  Operator=pow  SignedPower=on
  Math Function4 : Math  Operator=pow  SignedPower=on
  Memory : Memory  InitialCondition=0.1
  N(rpm) : Product  Inputs=*/
  N(rpm)1 : Product  Inputs=/*
  P Scope : Scope  NumInputPorts=2
  P_sp : Product  Inputs=4
  Product1 : Product
  Product2 : Product
  Q : Product  Inputs=4
  RPM 2 : Scope
  Saturation : Saturate  UpperLimit=104.72  LowerLimit=0.1
  Scope : Scope
  Sum : Sum  Inputs=|+-
  Ueo : Product
  Um : Sum  Inputs=+-
  get CP : Lookup_n-D  BreakpointsForDimension1=Prop.J  BreakpointsForDimension2=Prop.theta_b  IndexSearchMethod=Linear search  BeginIndexSearchUsingPreviousIndexResult=on  Table=Prop.CP  RndMeth=Simplest
      settings: InputPortMap=u0,u1
  "n^3 " : Constant  Value=3
  rpm : Outport  VectorParamsAs1DForOutWhenUnconnected=off
  wires:
  Saturation/1 -> Gain1/1, Divide/2
  Gain2/1 -> Integrator/2
  rpm0/1 -> Manual Switch/1
  Gain1/1 -> rpm/1, RPM 2/1  "rpm"
  Sum/1 -> Divide/1  "DP"
  Divide/1 -> Integrator/1  "omega_dot"
  dt/1 -> Ueo/1
  Integrator/1 -> Saturation/1  "omega"
  P_sp/1 -> Scope/1, P Scope/1, Sum/1
  P_shaft/1 -> P Scope/2, Sum/2
  Ix/1 -> Divide/3
  Constant/1 -> Ueo/2
  Ueo/1 -> Um/1
  Product1/1 -> Um/2
  Constant1/1 -> Product1/1
  Um/1 -> Ea/1
  Product2/1 -> Ea/2
  Constant2/1 -> Product2/1
  Ea/1 -> N(rpm)/1
  Constant3/1 -> N(rpm)/2
  Diameter/1 -> J/2
  V/1 -> J/1
  N(rpm)/1 -> Gain3/1
  J/1 -> get CP/1
  theta_b/1 -> get CP/2
  Gain4/1 -> Q/2  "CQ"
  D^5/1 -> Math Function4/2
  Diameter1/1 -> Math Function4/1
  Math Function/1 -> Q/3  "n^2"
  Q/1 -> N(rpm)1/2
  Constant4/1 -> N(rpm)1/1
  N(rpm)1/1 -> Im/1
  Constant5/1 -> Im/2
  Im/1 -> Product2/2, Product1/2
  rho/1 -> Q/1, P_sp/3  "rho"
  Math Function3/1 -> P_sp/2  "n^3"
  "n^3 "/1 -> Math Function3/2
  Math Function4/1 -> Q/4, P_sp/4  "D^5"
  get CP/1 -> Gain4/1, P_sp/1  "CP"
  Constant6/1 -> Manual Switch/2
  Manual Switch/1 -> Gain2/1
  Gain3/1 -> Memory/1  "rps"
  Memory/1 -> J/3, Math Function3/1, Math Function/1

== system eVTOL_PX4_2023b/Subsystem1/Energy & Power/thrust_2/Propeller  ==
  rpm : Inport
  V : Inport  Port=2
  rho : Inport  Port=3
  theta_b : Inport  Port=4
  D^5 : Constant  Value=5
  Diameter : Constant  Value=Prop.D
  Divide : Product  Inputs=4
  Divide2 : Product  Inputs=4
  Divide3 : Product  Inputs=**/
  Gain : Gain  Gain=1/60
  Math Function : Math  Operator=magnitude^2  SignedPower=on
  Math Function1 : Math  Operator=magnitude^2  SignedPower=on
  Math Function2 : Math  Operator=magnitude^2  SignedPower=on
  Math Function3 : Math  Operator=pow  SignedPower=on
  Math Function4 : Math  Operator=pow  SignedPower=on
  Scope{,1..4} (5 alike) : Scope
  Subsystem : Subsystem
  get CP : Lookup_n-D  BreakpointsForDimension1=Prop.J  BreakpointsForDimension2=Prop.theta_b  IndexSearchMethod=Linear search  BeginIndexSearchUsingPreviousIndexResult=on  Table=Prop.CP  RndMeth=Simplest
      settings: InputPortMap=u0,u1
  get CT : Lookup_n-D  BreakpointsForDimension1=Prop.J  BreakpointsForDimension2=Prop.theta_b  IndexSearchMethod=Linear search  BeginIndexSearchUsingPreviousIndexResult=on  Table=Prop.CT  RndMeth=Simplest
      settings: InputPortMap=u0,u1
  "n^3 " : Constant  Value=3
  P_plr (w) : Outport  VectorParamsAs1DForOutWhenUnconnected=off
  T (N) : Outport  Port=2  VectorParamsAs1DForOutWhenUnconnected=off
  eta_p : Outport  Port=3  VectorParamsAs1DForOutWhenUnconnected=off
  wires:
  Divide2/1 -> P_plr (w)/1, Scope/1
  Divide3/1 -> eta_p/1  "eta_p"
  D^5/1 -> Math Function4/2
  Math Function4/1 -> Divide2/4
  "n^3 "/1 -> Math Function3/2
  Math Function3/1 -> Divide2/3
  get CP/1 -> Divide3/3, Divide2/1, Scope3/1
  rpm/1 -> Gain/1, Subsystem/2(rpm)
  Subsystem/1(J) -> Scope2/1, get CT/1, Divide3/1, get CP/1
  Divide/1 -> Scope1/1, T (N)/1
  Math Function2/1 -> Divide/4  "D^4"
  Math Function1/1 -> Math Function2/1
  Diameter/1 -> Math Function1/1, Math Function4/1
  Math Function/1 -> Divide/3  "n^2"
  Gain/1 -> Math Function3/1, Math Function/1
  rho/1 -> Divide/2, Divide2/2
  get CT/1 -> Divide3/2, Divide/1, Scope4/1
  V/1 -> Subsystem/1(V)
  theta_b/1 -> get CP/2, get CT/2
